simulink model "respuestas_continuo"  (R2024a)
settings: Solver=VariableStepAuto  StartTime=0.0  StopTime=200  RelTol=1e-3
libraries: fuzblock x1
settings Model: Creator=MSI  LastModifiedBy=USER
settings RTWCC: GPUComputeCapability=3.5

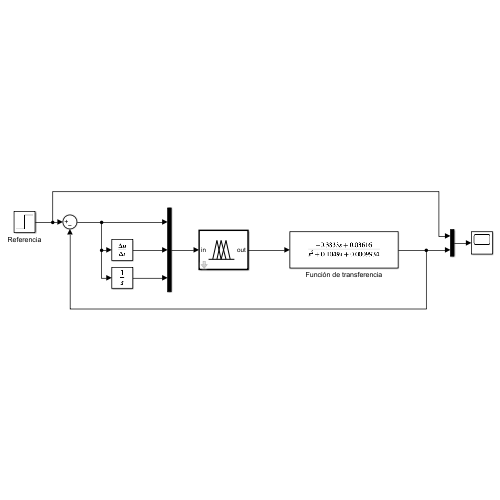
[thumbnail: Simulink's stored preview of the top-level diagram]
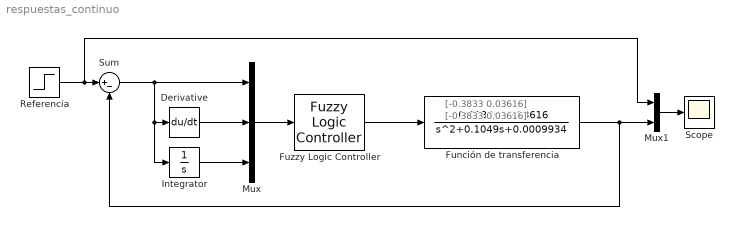
== system respuestas_continuo ==
  note: [-0.3833 0.03616]
  note: [-0.3833 0.03616]
  Derivative : Derivative
  Función de transferencia : TransferFcn  Numerator="[-0.3833  0.03616]"  Denominator=[1 0.1049 0.0009934]
  Fuzzy Logic Controller : fuzblock/Fuzzy Logic  Controller  FIS='planta_fuzzy.fis'  OutputSampleNumber=101  DataType=double  FuzzifiedInputs=off  RuleFiringStrengths=off  RuleOutputs=off  AggregatedOutputs=off  SimulateUsing=Interpreted execution  OutOfRangeInputValueMessage=warning  NoRuleFiredMessage=warning  EmptyOutputFuzzySetMessage=warning
  Integrator : Integrator
  Mux : Mux  Inputs=3
  Mux1 : Mux  Inputs=2
  Referencia : Step  After=30  SampleTime=0
  Scope : Scope
  Sum : Sum  Inputs=|+-
  wires:
  Sum/1 -> Mux/1, Integrator/1, Derivative/1
  Derivative/1 -> Mux/2
  Integrator/1 -> Mux/3
  Mux/1 -> Fuzzy Logic Controller/1
  Fuzzy Logic Controller/1 -> Función de transferencia/1
  Referencia/1 -> Mux1/1, Sum/1
  Función de transferencia/1 -> Mux1/2, Sum/2
  Mux1/1 -> Scope/1
